simulink model "ueb1_2"  (R2013a)
settings: Solver=ode45  StartTime=0.0  StopTime=10.0  RelTol=1e-3
values from neighbouring files (symbols this model uses):
  c1 = 9*10^4    (= 90000)    [Script1_2e.m]    (also in balken_analytisch.m = u_quer/(2*l*alpha) * ( (l-b)^2 - (l-a)^2 ))
  c2 = 3*10^4    (= 30000)    [Script1_2e.m]    (also in balken_analytisch.m = 0)
  d2 = 750    [Script1_2e.m]
  m1 = 25    [Script1_2e.m]
  m2 = 250    [Script1_2e.m]
settings Model: Creator=isyssim2  LastModifiedBy=isyssim2

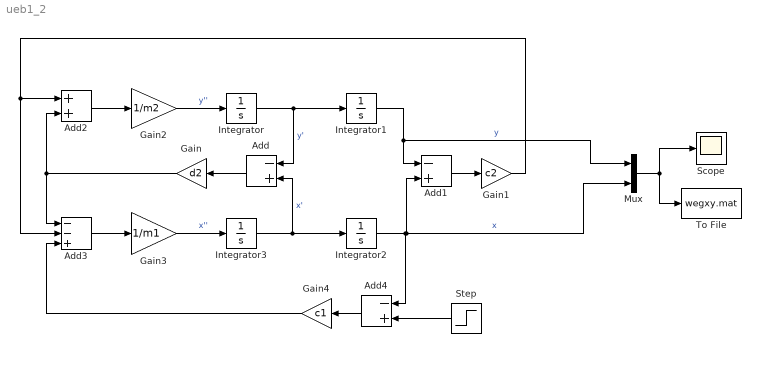
== system ueb1_2 ==
  Add : Sum  Inputs=-+
  Add1 : Sum  Inputs=-+
  Add2 : Sum
  Add3 : Sum  Inputs=--+
  Add4 : Sum  Inputs=-+
  Gain : Gain  Gain=d2
  Gain1 : Gain  Gain=c2
  Gain2 : Gain  Gain=1/m2
  Gain3 : Gain  Gain=1/m1
  Gain4 : Gain  Gain=c1
  Integrator{,1..3} (4 alike) : Integrator
  Mux : Mux  Inputs=2
  Scope : Scope
  Step : Step  SampleTime=0
  To File : ToFile  Filename=wegxy.mat
  wires:
  Integrator3/1 -> Add/2, Integrator2/1  "x'"
  Integrator/1 -> Add/1, Integrator1/1  "y'"
  Integrator1/1 -> Mux/1, Add1/1  "y"
  Integrator2/1 -> Mux/2, Add1/2, Add4/1  "x"
  Gain2/1 -> Integrator/1  "y''"
  Gain3/1 -> Integrator3/1  "x''"
  Add/1 -> Gain/1
  Add1/1 -> Gain1/1
  Add2/1 -> Gain2/1
  Gain1/1 -> Add3/2, Add2/1
  Gain/1 -> Add2/2, Add3/1
  Add3/1 -> Gain3/1
  Step/1 -> Add4/2
  Add4/1 -> Gain4/1
  Gain4/1 -> Add3/3
  Mux/1 -> To File/1, Scope/1
